simulink model "uart_xy_wiggler"  (R2018a)
settings: Solver=FixedStepDiscrete  StartTime=0.0  StopTime=inf  RelTol=1e-3
PreLoadFcn:
  | waijung.modelPreload; % Required for working with Waijung Blockset. Do not remove.
undefined symbols (not defined in the file or in its folder): HSEOSC, Link, LQFP144, ST, STM32F446ZE
libraries: simulink x10, commsynccomp2 x7, stm32f4_io_lib x3, dspstat3 x2, stm32f4_device_config_lib x1, dspbuff3 x1
(part 3 of 9)

== system uart_xy_wiggler/Lissajous Data ==
  Volatile Data Storage10 : S-Function  FunctionName=waijung_vdata_storage  Parameters=storagetype,storagename,initval,varname,buffersize,initvalstring,sampletime,sampletimestr,blockid,storagetypestr  SFunctionDeploymentMode=off  EnableBusSupport=off  mask(waijung_vdata_storage){storagetype=double, definevolatile=on, storagename=Ays, initval=1, varname=LissajousDataVolatileDataStorage10_Ays, buffersize=64, initvalstring='Initial string', webintegration=Disable, weboutputformat='%f', webcgicallback=(void*)0, laststoragetype=double, sampletime=-1, sampletimestr=-1, blockid=LissajousDataVolatileDataStorage10, storagetypestr=volatile double}
      mask prompts: storagetype "Storage Type"; definevolatile "Define with "volatile" keyword"; storagename "Storage Name (must be a valid variable name)"; initval "Initial value (Apply at Power on Reset only)"; varname "Variable name"; buffersize "Size (bytes)"; initvalstring "Initial value (Apply at Power on Reset only)"; webintegration "Web CGI varget/varset integration"; weboutputformat "Web CGI varget output format"; webcgicallback "Web CGI varset callback"; laststoragetype "Last selected Storage Type"; sampletime "Sample time (sec)"; sampletimestr "Compiled sample time (sec) in string"; storagetypestr "Type string"
      mask help:
      | This block implements a volatile Data Storage.
      |
      | Web CGI varset/varget integratiopn:
      | Enable - In webserver application, allow remote access via http.
      | Disable - Variable is use in local only.
      mask init:
      | waijung_vdata_storage_callback('init');
      mask Help: web(fullfile(waijungdocroot,'Volatile_Data_Storage.htm'))
      mask TypeOptions storagetype: double | single | uint32 | int32 | uint16 | int16 | uint8 | int8 | string
      mask Callback storagetype: waijung_vdata_storage_callback('storagetype');
      mask Callback storagename: waijung_vdata_storage_callback('storagename');
      mask Callback initval: waijung_vdata_storage_callback('initval');
      mask Callback varname: waijung_vdata_storage_callback('varname');
      mask Callback initvalstring: waijung_vdata_storage_callback('initvalstring');
      mask TypeOptions webintegration: Disable | ReadOnly | Write/ Read | ReadOnly with KeyValuePair | Write/ Read with KeyValuePair
      mask Callback webintegration: waijung_vdata_storage_callback('webintegration');
      mask Callback weboutputformat: waijung_vdata_storage_callback('weboutputformat');
      mask TypeOptions laststoragetype: double | single | uint32 | int32 | uint16 | int16 | uint8 | int8 | string
      mask Callback sampletime: waijung_vdata_storage_callback('sampletime');
      mask Callback sampletimestr: waijung_vdata_storage_callback('sampletimestr');
      mask Callback blockid: waijung_vdata_storage_callback('blockid');
      mask Display: text(0.5, 0.5, 'Name: Ays\nType: double','ver','middle','hor','center')
  Volatile Data Storage11 : S-Function  FunctionName=waijung_vdata_storage  Parameters=storagetype,storagename,initval,varname,buffersize,initvalstring,sampletime,sampletimestr,blockid,storagetypestr  SFunctionDeploymentMode=off  EnableBusSupport=off  mask(waijung_vdata_storage){storagetype=double, definevolatile=on, storagename=Ayc, initval=1, varname=LissajousDataVolatileDataStorage11_Ayc, buffersize=64, initvalstring='Initial string', webintegration=Disable, weboutputformat='%f', webcgicallback=(void*)0, laststoragetype=double, sampletime=-1, sampletimestr=-1, blockid=LissajousDataVolatileDataStorage11, storagetypestr=volatile double}
      mask prompts: storagetype "Storage Type"; definevolatile "Define with "volatile" keyword"; storagename "Storage Name (must be a valid variable name)"; initval "Initial value (Apply at Power on Reset only)"; varname "Variable name"; buffersize "Size (bytes)"; initvalstring "Initial value (Apply at Power on Reset only)"; webintegration "Web CGI varget/varset integration"; weboutputformat "Web CGI varget output format"; webcgicallback "Web CGI varset callback"; laststoragetype "Last selected Storage Type"; sampletime "Sample time (sec)"; sampletimestr "Compiled sample time (sec) in string"; storagetypestr "Type string"
      mask help:
      | This block implements a volatile Data Storage.
      |
      | Web CGI varset/varget integratiopn:
      | Enable - In webserver application, allow remote access via http.
      | Disable - Variable is use in local only.
      mask init:
      | waijung_vdata_storage_callback('init');
      mask Help: web(fullfile(waijungdocroot,'Volatile_Data_Storage.htm'))
      mask TypeOptions storagetype: double | single | uint32 | int32 | uint16 | int16 | uint8 | int8 | string
      mask Callback storagetype: waijung_vdata_storage_callback('storagetype');
      mask Callback storagename: waijung_vdata_storage_callback('storagename');
      mask Callback initval: waijung_vdata_storage_callback('initval');
      mask Callback varname: waijung_vdata_storage_callback('varname');
      mask Callback initvalstring: waijung_vdata_storage_callback('initvalstring');
      mask TypeOptions webintegration: Disable | ReadOnly | Write/ Read | ReadOnly with KeyValuePair | Write/ Read with KeyValuePair
      mask Callback webintegration: waijung_vdata_storage_callback('webintegration');
      mask Callback weboutputformat: waijung_vdata_storage_callback('weboutputformat');
      mask TypeOptions laststoragetype: double | single | uint32 | int32 | uint16 | int16 | uint8 | int8 | string
      mask Callback sampletime: waijung_vdata_storage_callback('sampletime');
      mask Callback sampletimestr: waijung_vdata_storage_callback('sampletimestr');
      mask Callback blockid: waijung_vdata_storage_callback('blockid');
      mask Display: text(0.5, 0.5, 'Name: Ayc\nType: double','ver','middle','hor','center')
  Volatile Data Storage12 : S-Function  FunctionName=waijung_vdata_storage  Parameters=storagetype,storagename,initval,varname,buffersize,initvalstring,sampletime,sampletimestr,blockid,storagetypestr  SFunctionDeploymentMode=off  EnableBusSupport=off  mask(waijung_vdata_storage){storagetype=double, definevolatile=on, storagename=Axs, initval=1, varname=LissajousDataVolatileDataStorage12_Axs, buffersize=64, initvalstring='Initial string', webintegration=Disable, weboutputformat='%f', webcgicallback=(void*)0, laststoragetype=double, sampletime=-1, sampletimestr=-1, blockid=LissajousDataVolatileDataStorage12, storagetypestr=volatile double}
      mask prompts: storagetype "Storage Type"; definevolatile "Define with "volatile" keyword"; storagename "Storage Name (must be a valid variable name)"; initval "Initial value (Apply at Power on Reset only)"; varname "Variable name"; buffersize "Size (bytes)"; initvalstring "Initial value (Apply at Power on Reset only)"; webintegration "Web CGI varget/varset integration"; weboutputformat "Web CGI varget output format"; webcgicallback "Web CGI varset callback"; laststoragetype "Last selected Storage Type"; sampletime "Sample time (sec)"; sampletimestr "Compiled sample time (sec) in string"; storagetypestr "Type string"
      mask help:
      | This block implements a volatile Data Storage.
      |
      | Web CGI varset/varget integratiopn:
      | Enable - In webserver application, allow remote access via http.
      | Disable - Variable is use in local only.
      mask init:
      | waijung_vdata_storage_callback('init');
      mask Help: web(fullfile(waijungdocroot,'Volatile_Data_Storage.htm'))
      mask TypeOptions storagetype: double | single | uint32 | int32 | uint16 | int16 | uint8 | int8 | string
      mask Callback storagetype: waijung_vdata_storage_callback('storagetype');
      mask Callback storagename: waijung_vdata_storage_callback('storagename');
      mask Callback initval: waijung_vdata_storage_callback('initval');
      mask Callback varname: waijung_vdata_storage_callback('varname');
      mask Callback initvalstring: waijung_vdata_storage_callback('initvalstring');
      mask TypeOptions webintegration: Disable | ReadOnly | Write/ Read | ReadOnly with KeyValuePair | Write/ Read with KeyValuePair
      mask Callback webintegration: waijung_vdata_storage_callback('webintegration');
      mask Callback weboutputformat: waijung_vdata_storage_callback('weboutputformat');
      mask TypeOptions laststoragetype: double | single | uint32 | int32 | uint16 | int16 | uint8 | int8 | string
      mask Callback sampletime: waijung_vdata_storage_callback('sampletime');
      mask Callback sampletimestr: waijung_vdata_storage_callback('sampletimestr');
      mask Callback blockid: waijung_vdata_storage_callback('blockid');
      mask Display: text(0.5, 0.5, 'Name: Axs\nType: double','ver','middle','hor','center')
  Volatile Data Storage7 : S-Function  FunctionName=waijung_vdata_storage  Parameters=storagetype,storagename,initval,varname,buffersize,initvalstring,sampletime,sampletimestr,blockid,storagetypestr  SFunctionDeploymentMode=off  EnableBusSupport=off  mask(waijung_vdata_storage){storagetype=double, definevolatile=on, storagename=A_Laser, initval=0.1, varname=LissajousDataVolatileDataStorage7_A_Laser, buffersize=64, initvalstring='Initial string', webintegration=Disable, weboutputformat='%f', webcgicallback=(void*)0, laststoragetype=double, sampletime=-1, sampletimestr=-1, blockid=LissajousDataVolatileDataStorage7, storagetypestr=volatile double}
      mask prompts: storagetype "Storage Type"; definevolatile "Define with "volatile" keyword"; storagename "Storage Name (must be a valid variable name)"; initval "Initial value (Apply at Power on Reset only)"; varname "Variable name"; buffersize "Size (bytes)"; initvalstring "Initial value (Apply at Power on Reset only)"; webintegration "Web CGI varget/varset integration"; weboutputformat "Web CGI varget output format"; webcgicallback "Web CGI varset callback"; laststoragetype "Last selected Storage Type"; sampletime "Sample time (sec)"; sampletimestr "Compiled sample time (sec) in string"; storagetypestr "Type string"
      mask help:
      | This block implements a volatile Data Storage.
      |
      | Web CGI varset/varget integratiopn:
      | Enable - In webserver application, allow remote access via http.
      | Disable - Variable is use in local only.
      mask init:
      | waijung_vdata_storage_callback('init');
      mask Help: web(fullfile(waijungdocroot,'Volatile_Data_Storage.htm'))
      mask TypeOptions storagetype: double | single | uint32 | int32 | uint16 | int16 | uint8 | int8 | string
      mask Callback storagetype: waijung_vdata_storage_callback('storagetype');
      mask Callback storagename: waijung_vdata_storage_callback('storagename');
      mask Callback initval: waijung_vdata_storage_callback('initval');
      mask Callback varname: waijung_vdata_storage_callback('varname');
      mask Callback initvalstring: waijung_vdata_storage_callback('initvalstring');
      mask TypeOptions webintegration: Disable | ReadOnly | Write/ Read | ReadOnly with KeyValuePair | Write/ Read with KeyValuePair
      mask Callback webintegration: waijung_vdata_storage_callback('webintegration');
      mask Callback weboutputformat: waijung_vdata_storage_callback('weboutputformat');
      mask TypeOptions laststoragetype: double | single | uint32 | int32 | uint16 | int16 | uint8 | int8 | string
      mask Callback sampletime: waijung_vdata_storage_callback('sampletime');
      mask Callback sampletimestr: waijung_vdata_storage_callback('sampletimestr');
      mask Callback blockid: waijung_vdata_storage_callback('blockid');
      mask Display: text(0.5, 0.5, 'Name: A_Laser\nType: double','ver','middle','hor','center')
  Volatile Data Storage8 : S-Function  FunctionName=waijung_vdata_storage  Parameters=storagetype,storagename,initval,varname,buffersize,initvalstring,sampletime,sampletimestr,blockid,storagetypestr  SFunctionDeploymentMode=off  EnableBusSupport=off  mask(waijung_vdata_storage){storagetype=double, definevolatile=on, storagename=LissaFreq, initval=0.1, varname=LissajousDataVolatileDataStorage8_LissaFreq, buffersize=64, initvalstring='Initial string', webintegration=Disable, weboutputformat='%f', webcgicallback=(void*)0, laststoragetype=double, sampletime=-1, sampletimestr=-1, blockid=LissajousDataVolatileDataStorage8, storagetypestr=volatile double}
      mask prompts: storagetype "Storage Type"; definevolatile "Define with "volatile" keyword"; storagename "Storage Name (must be a valid variable name)"; initval "Initial value (Apply at Power on Reset only)"; varname "Variable name"; buffersize "Size (bytes)"; initvalstring "Initial value (Apply at Power on Reset only)"; webintegration "Web CGI varget/varset integration"; weboutputformat "Web CGI varget output format"; webcgicallback "Web CGI varset callback"; laststoragetype "Last selected Storage Type"; sampletime "Sample time (sec)"; sampletimestr "Compiled sample time (sec) in string"; storagetypestr "Type string"
      mask help:
      | This block implements a volatile Data Storage.
      |
      | Web CGI varset/varget integratiopn:
      | Enable - In webserver application, allow remote access via http.
      | Disable - Variable is use in local only.
      mask init:
      | waijung_vdata_storage_callback('init');
      mask Help: web(fullfile(waijungdocroot,'Volatile_Data_Storage.htm'))
      mask TypeOptions storagetype: double | single | uint32 | int32 | uint16 | int16 | uint8 | int8 | string
      mask Callback storagetype: waijung_vdata_storage_callback('storagetype');
      mask Callback storagename: waijung_vdata_storage_callback('storagename');
      mask Callback initval: waijung_vdata_storage_callback('initval');
      mask Callback varname: waijung_vdata_storage_callback('varname');
      mask Callback initvalstring: waijung_vdata_storage_callback('initvalstring');
      mask TypeOptions webintegration: Disable | ReadOnly | Write/ Read | ReadOnly with KeyValuePair | Write/ Read with KeyValuePair
      mask Callback webintegration: waijung_vdata_storage_callback('webintegration');
      mask Callback weboutputformat: waijung_vdata_storage_callback('weboutputformat');
      mask TypeOptions laststoragetype: double | single | uint32 | int32 | uint16 | int16 | uint8 | int8 | string
      mask Callback sampletime: waijung_vdata_storage_callback('sampletime');
      mask Callback sampletimestr: waijung_vdata_storage_callback('sampletimestr');
      mask Callback blockid: waijung_vdata_storage_callback('blockid');
      mask Display: text(0.5, 0.5, 'Name: LissaFreq\nType: double','ver','middle','hor','center')
  Volatile Data Storage9 : S-Function  FunctionName=waijung_vdata_storage  Parameters=storagetype,storagename,initval,varname,buffersize,initvalstring,sampletime,sampletimestr,blockid,storagetypestr  SFunctionDeploymentMode=off  EnableBusSupport=off  mask(waijung_vdata_storage){storagetype=double, definevolatile=on, storagename=Axc, initval=1, varname=LissajousDataVolatileDataStorage9_Axc, buffersize=64, initvalstring='Initial string', webintegration=Disable, weboutputformat='%f', webcgicallback=(void*)0, laststoragetype=double, sampletime=-1, sampletimestr=-1, blockid=LissajousDataVolatileDataStorage9, storagetypestr=volatile double}
      mask prompts: storagetype "Storage Type"; definevolatile "Define with "volatile" keyword"; storagename "Storage Name (must be a valid variable name)"; initval "Initial value (Apply at Power on Reset only)"; varname "Variable name"; buffersize "Size (bytes)"; initvalstring "Initial value (Apply at Power on Reset only)"; webintegration "Web CGI varget/varset integration"; weboutputformat "Web CGI varget output format"; webcgicallback "Web CGI varset callback"; laststoragetype "Last selected Storage Type"; sampletime "Sample time (sec)"; sampletimestr "Compiled sample time (sec) in string"; storagetypestr "Type string"
      mask help:
      | This block implements a volatile Data Storage.
      |
      | Web CGI varset/varget integratiopn:
      | Enable - In webserver application, allow remote access via http.
      | Disable - Variable is use in local only.
      mask init:
      | waijung_vdata_storage_callback('init');
      mask Help: web(fullfile(waijungdocroot,'Volatile_Data_Storage.htm'))
      mask TypeOptions storagetype: double | single | uint32 | int32 | uint16 | int16 | uint8 | int8 | string
      mask Callback storagetype: waijung_vdata_storage_callback('storagetype');
      mask Callback storagename: waijung_vdata_storage_callback('storagename');
      mask Callback initval: waijung_vdata_storage_callback('initval');
      mask Callback varname: waijung_vdata_storage_callback('varname');
      mask Callback initvalstring: waijung_vdata_storage_callback('initvalstring');
      mask TypeOptions webintegration: Disable | ReadOnly | Write/ Read | ReadOnly with KeyValuePair | Write/ Read with KeyValuePair
      mask Callback webintegration: waijung_vdata_storage_callback('webintegration');
      mask Callback weboutputformat: waijung_vdata_storage_callback('weboutputformat');
      mask TypeOptions laststoragetype: double | single | uint32 | int32 | uint16 | int16 | uint8 | int8 | string
      mask Callback sampletime: waijung_vdata_storage_callback('sampletime');
      mask Callback sampletimestr: waijung_vdata_storage_callback('sampletimestr');
      mask Callback blockid: waijung_vdata_storage_callback('blockid');
      mask Display: text(0.5, 0.5, 'Name: Axc\nType: double','ver','middle','hor','center')

== system uart_xy_wiggler/UART_parameter_input ==

== system uart_xy_wiggler/ignore_bad_data ==
  ADXL_X : Inport
  Compare To Constant10 : simulink/Logic and Bit Operations/Compare To Constant  relop=>  const=-50  OutDataTypeStr=boolean
  Compare To Constant8 : simulink/Logic and Bit Operations/Compare To Constant  relop=<  const=50  OutDataTypeStr=boolean
  Delay2 : Delay  DelayLength=1
  Logical Operator4 : Logic  AllPortsSameDT=off  OutDataTypeStr=boolean
  Switch2 : Switch  Criteria=u2 > Threshold
  Out1 : Outport
  wires:
  Compare To Constant10/1 -> Logical Operator4/2
  Logical Operator4/1 -> Switch2/2
  Switch2/1 -> Delay2/1, Out1/1
  ADXL_X/1 -> Switch2/1, Compare To Constant8/1, Compare To Constant10/1
  Compare To Constant8/1 -> Logical Operator4/1
  Delay2/1 -> Switch2/3

== system uart_xy_wiggler/ignore_bad_data1 ==
  ADXL_X : Inport
  Compare To Constant10 : simulink/Logic and Bit Operations/Compare To Constant  relop=>  const=-50  OutDataTypeStr=boolean
  Compare To Constant8 : simulink/Logic and Bit Operations/Compare To Constant  relop=<  const=50  OutDataTypeStr=boolean
  Delay2 : Delay  DelayLength=1
  Logical Operator4 : Logic  AllPortsSameDT=off  OutDataTypeStr=boolean
  Switch2 : Switch  Criteria=u2 > Threshold
  Out1 : Outport
  wires:
  Delay2/1 -> Switch2/3
  Compare To Constant8/1 -> Logical Operator4/1
  ADXL_X/1 -> Compare To Constant10/1, Compare To Constant8/1, Switch2/1
  Switch2/1 -> Out1/1, Delay2/1
  Logical Operator4/1 -> Switch2/2
  Compare To Constant10/1 -> Logical Operator4/2

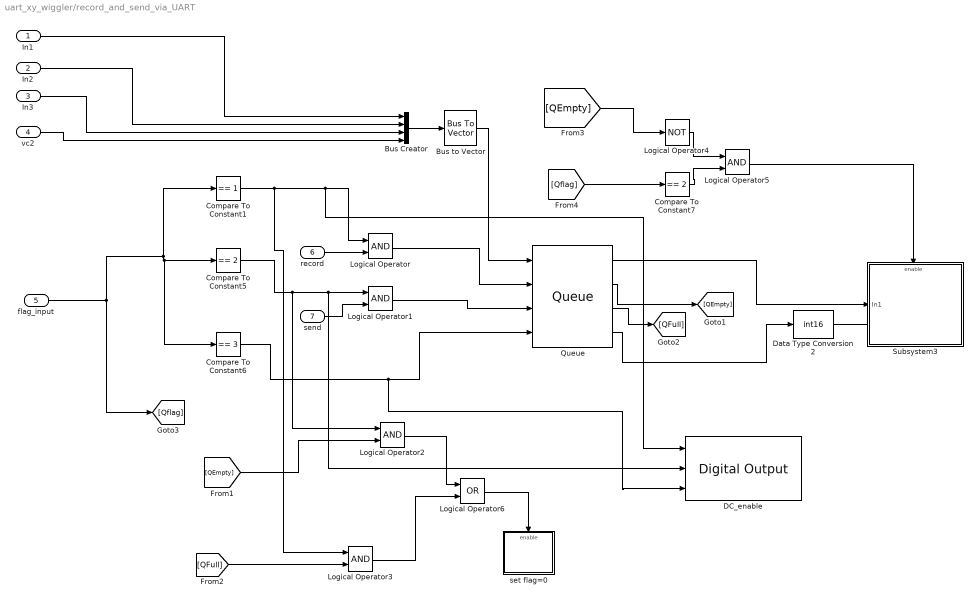
== system uart_xy_wiggler/record_and_send_via_UART ==
  In1 : Inport
  In2 : Inport  Port=2
  In3 : Inport  Port=3
  vc2 : Inport  Port=4
  flag_input : Inport  Port=5
  record : Inport  Port=6
  send : Inport  Port=7
  Bus Creator : BusCreator  Inputs=4
  Bus to Vector : BusToVector
  Compare To Constant1 : simulink/Logic and Bit Operations/Compare To Constant  relop===  const=1  OutDataTypeStr=boolean
  Compare To Constant5 : simulink/Logic and Bit Operations/Compare To Constant  relop===  const=2  OutDataTypeStr=boolean
  Compare To Constant6 : simulink/Logic and Bit Operations/Compare To Constant  relop===  const=3  OutDataTypeStr=boolean
  Compare To Constant7 : simulink/Logic and Bit Operations/Compare To Constant  relop===  const=2  OutDataTypeStr=boolean
  DC_enable : stm32f4_io_lib/Digital Output  use_bitband=on  port=B  speed=100  porttype=Push Pull  porttypestr=PP  use_pin0=on  use_pin1=off  use_pin2=off  use_pin3=off  use_pin4=off  use_pin5=off  use_pin6=off  use_pin7=on  use_pin8=off  use_pin9=off  use_pin10=off  use_pin11=off  use_pin12=off  use_pin13=off  use_pin14=on  use_pin15=off  pinstr=GPIO_Pin_0 | GPIO_Pin_7 | GPIO_Pin_14  usedpinarray="[1  0  0  0  0  0  0  1  0  0  0  0  0  0  1  0]"  bitbandingstr=|  sampletime=-1  sampletimestr=-1  blockid=record_and_send_via_UARTDC_enable  enablecustomportlabel=off  globalinit=off  cinputportlabel=In1, In2  coutputportlabel=0
      | #define record_and_send_via_UARTDC_enable_B0 Peripheral_BB(GPIOB->ODR, 0)  /* Output pin */
      | #define record_and_send_via_UARTDC_enable_B7 Peripheral_BB(GPIOB->ODR, 7)  /* Output pin */
      | #define record_and_send_via_UARTDC_enable_B14 Peripheral_BB(GPIOB->ODR, 14)  /* Output pin */
      settings: SourceProductName=Waijung Blockset
  Data Type Conversion2 : DataTypeConversion  OutDataTypeStr=int16
  Logical Operator{,1..3,5} (5 alike) : Logic  AllPortsSameDT=off  OutDataTypeStr=boolean
  Logical Operator4 : Logic  Operator=NOT  AllPortsSameDT=off  OutDataTypeStr=boolean
  Logical Operator6 : Logic  Operator=OR  AllPortsSameDT=off  OutDataTypeStr=boolean
  Queue : dspbuff3/Queue  depth=20  trigger=Either edge  overflow=Ignore  pes=Ignore  eso=on  fso=on  nso=on  clr=on  clrOutport=on  adf=on
      settings: SourceProductName=DSP System Toolbox  SourceProductBaseCode=DS
  Subsystem3 : Subsystem
  set flag=0 : Subsystem
  wires:
  send/1 -> Logical Operator1/2
  [QFull] -> Logical Operator3/2
  Queue/4 -> Data Type Conversion2/1
  Logical Operator/1 -> Queue/2
  record/1 -> Logical Operator/2
  Logical Operator1/1 -> Queue/3
  Queue/2 -> [QEmpty]
  Logical Operator3/1 -> Logical Operator6/2
  Compare To Constant7/1 -> Logical Operator5/2
  Compare To Constant5/1 -> DC_enable/2, Logical Operator1/1, Logical Operator2/1
  Compare To Constant1/1 -> Logical Operator3/1, DC_enable/1, Logical Operator/1
  [QEmpty] -> Logical Operator2/2
  Compare To Constant6/1 -> DC_enable/3, Queue/4
  [QEmpty] -> Logical Operator4/1
  Logical Operator4/1 -> Logical Operator5/1
  Queue/3 -> [QFull]
  [Qflag] -> Compare To Constant7/1
  Logical Operator5/1 -> Subsystem3/Enable
  Logical Operator6/1 -> set flag=0/Enable
  Bus Creator/1 -> Bus to Vector/1
  Bus to Vector/1 -> Queue/1
  In2/1 -> Bus Creator/2
  Logical Operator2/1 -> Logical Operator6/1
  In1/1 -> Bus Creator/1
  Queue/1 -> Subsystem3/1(In1)
  flag_input/1 -> [Qflag], Compare To Constant6/1, Compare To Constant5/1, Compare To Constant1/1
  Data Type Conversion2/1 -> ?
  In3/1 -> Bus Creator/3
  vc2/1 -> Bus Creator/4
